simulink model "LaneFollowingNMPC"  (R2021a)
settings: Solver=FixedStepAuto  StartTime=0.0  StopTime=t(end)  FixedStep=Ts  RelTol=1e-3
PreLoadFcn:
  | LaneFollowingUsingNMPCData
values from neighbouring files (symbols this model uses):
  nlobj = nlmpc(7,3,'MV',[1 2],'MD',3,'UD',4)    [LaneFollowingUsingNMPCExample.m]
  phi0 = 0    [CurriculumAngledGetCurvature.m]    (also in DoubleLaneChangeGetCurvature.m; FalconeDoubleLaneChangeGetCurvature.m; FigureEightGetCurvature.m = 1.57079632679; HairpinGetCurvature.m = 1.57079632679)
  Ts = u(5)    [LaneFollowingEKFStateFcn.m]    (also in LaneFollowingUsingNMPCData.m = 0.05; read_csv_model.m = 0.05)
  v0 = v_seq_1.signals.values(1)    [LaneFollowingUsingNMPCData.m]
  v_seq = repelem(Vx, size(Xref, 2))    [FigureEightGetCurvature.m]    (also in LaneFollowingUsingNMPCData.m = v_seq_1.signals.values)
  Xref = [x_initial, Xref(1, 2:end)]    [CurriculumAngledGetCurvature.m]    (also in DoubleLaneChangeGetCurvature.m = Vx*time; FalconeDoubleLaneChangeGetCurvature.m = 0.0:0.05:120; FigureEightGetCurvature.m = A * cos(2. * pi * segments / num_segments); HairpinGetCurvature.m = [Xref, last_arm])
  Yref = [y_initial, Yref(1, 2:end)]    [CurriculumAngledGetCurvature.m]    (also in DoubleLaneChangeGetCurvature.m = 8.1/2*(1+tanh(z1)) - 11.4/2.*(1+tanh(z2)); FalconeDoubleLaneChangeGetCurvature.m = 4.05/2*(1+tanh(z1)) - 5.7/2.*(1+tanh(z2)); FigureEightGetCurvature.m = B * 0.5 * sin(4. * pi * segments / num_segments); HairpinGetCurvature.m = [Yref, last_arm_y])
undefined symbols (not defined in the file or in its folder): DiscIntNeverNeededParam, rho, v_seq_1
libraries: mpcadaslib x1, sharedTrackingLibrary x1, mpclib x1, autolibshared x1
settings Model: NumberOfSteps=3  Creator=The MathWorks, Inc.  LastModifiedBy=sarahaguasvivas
settings SolverCC: AlgebraicLoopSolver=TrustRegion
settings DataIOCC: ReturnWorkspaceOutputs=off
settings DebuggingCC: PregeneratedLibrarySubsystemCodeDiagnostic=none  SFMachineParentedDataDiag=warning  ArithmeticOperatorsInVariantConditions=warning
settings SFSimCC: SimUseLocalCustomCode=off  CustomCodeUndefinedFunction=UseInterfaceOnly
settings RTWCC: RTWUseLocalCustomCode=off
settings CodeAppCC: StateflowObjectComments=on

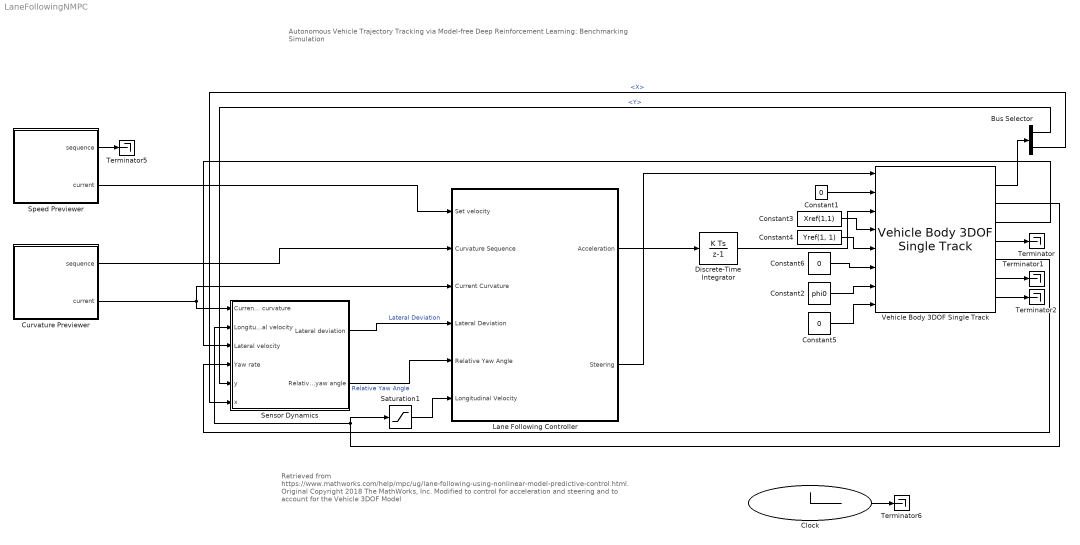
== system LaneFollowingNMPC ==
  note: Retrieved from https://www.mathworks.com/help/mpc/ug/lane-following-using-nonlinear-model-predictive-control.html. Original Copyright 2018 The MathWorks, Inc.
      |
      | Modified to control for acceleration and steering and to account for the Vehicle 3DOF Model
  note: Autonomous Vehicle Trajectory Tracking via Model-free Deep Reinforcement Learning: Benchmarking Simulation
  Bus Selector : BusSelector  OutputSignals=InertFrm.FrntAxl.Disp.Y,InertFrm.FrntAxl.Disp.X
  Clock : Clock
  Constant1 : Constant  Value=0
  Constant2 : Constant  Value=phi0
  Constant3 : Constant  Value=Xref(1,1)
  Constant4 : Constant  Value=Yref(1, 1)
  Constant5 : Constant  Value=0
  Constant6 : Constant  Value=0
  Curvature Previewer : Subsystem  mask{signal=rho, ts=Ts, steps=nlobj.PredictionHorizon}
      mask prompts: signal "Signal name"; ts "Sampling time"; steps "Number of previewing steps"
      mask init:
      | ts = evalin('base',get_param(gcbh,'ts'));
      | signal = evalin('base',get_param(gcbh,'signal'));
      | steps = evalin('base',get_param(gcbh,'steps'));
      | data = mpc_previewer_maskinit(signal,ts);
      mask Display:
      | fprintf('Future\nsample\nextractor');
      | port_label('output', 1, 'seq')
      | port_label('output', 2, '@t')
  Discrete-Time Integrator : DiscreteIntegrator  InitialCondition=v_seq(1)  SampleTime=Ts  LimitOutput=on  UpperSaturationLimit=50  ICPrevOutput=DiscIntNeverNeededParam  ICPrevScaledInput=DiscIntNeverNeededParam
  Lane Following Controller : Subsystem  Variant=on
  Saturation1 : Saturate  UpperLimit=Inf  LowerLimit=1e-5  OutDataTypeStr=double
  Sensor Dynamics : Subsystem
  Speed Previewer : Subsystem  mask{signal=v_seq_1, ts=Ts, steps=1}
      mask prompts: signal "Signal name"; ts "Sampling time"; steps "Number of previewing steps"
      mask init:
      | ts = evalin('base',get_param(gcbh,'ts'));
      | signal = evalin('base',get_param(gcbh,'signal'));
      | steps = evalin('base',get_param(gcbh,'steps'));
      | data = mpc_previewer_maskinit(signal,ts);
      mask Display:
      | fprintf('Future\nsample\nextractor');
      | port_label('output', 1, 'seq')
      | port_label('output', 2, '@t')
  Terminator{,1..2,5..6} (5 alike) : Terminator
  Vehicle Body 3DOF Single Track : autolibshared/Vehicle Body 3DOF Single Track  trackMode=Single (bicycle)  inputMode=External longitudinal velocity  frontSteerMode=on  rearSteerMode=on  windMode=off  muMode=off  extFMode=off  extMMode=off  htchFMode=off  htchMMode=off  extXo=on  extpsio=on  extxdoto=off  extro=on  extYo=on  extTamb=off  extydoto=on  aMode=2  NF=2  NR=2  m=2000  a=1.4  b=1.6  h=0.35  dh=1  hh=0.2  X_o=0  xdot_o=0  CalphaMode=off  sigmaMode=off  d=0  hl=0  w=[1.4,1.4]  Cy_f=19e3  Cy_r=33.5e3  sigma_f=.1  sigma_r=.1  alpha_f_brk=[-.1 .1]  Cy_f_data=[-9e3 9e3]  alpha_r_brk=[-.1 .1]  Cy_r_data=[-9e3 9e3]  Y_o=0  ydot_o=0  Izz=4000  psi_o=0  r_o=0  Af=0  Cd=.0  Cl=.0  Cpm=.0  beta_w=[0:0.01:0.3]  Cs=[0:0.03:0.9]  Cym=[0:0.01:0.3]  Pabs=101325  Tair=273  g=9.81  mu=1.  xdot_tol=.01  Fznom=5000  Fxtire_sat=7e4  Fytire_sat=7e4  longOff=0  latOff=0  vertOff=0  wrapAng=off
      settings: SourceProductBaseCode=PW,DR,MT,UV,VE
  wires:
  Vehicle Body 3DOF Single Track/5 -> Sensor Dynamics/4(Yaw rate)
  Sensor Dynamics/1(Lateral deviation) -> Lane Following Controller/4(Lateral Deviation)  "Lateral Deviation"
  Sensor Dynamics/2(Relative yaw angle) -> Lane Following Controller/5(Relative Yaw Angle)  "Relative Yaw Angle"
  Vehicle Body 3DOF Single Track/6 -> Terminator1/1
  Vehicle Body 3DOF Single Track/7 -> Terminator2/1
  Vehicle Body 3DOF Single Track/1 -> Bus Selector/1
  Vehicle Body 3DOF Single Track/3 -> Sensor Dynamics/3(Lateral velocity)
  Discrete-Time Integrator/1 -> Vehicle Body 3DOF Single Track/3
  Vehicle Body 3DOF Single Track/2 -> Saturation1/1, Sensor Dynamics/2(Longitudinal velocity)
  Speed Previewer/2(current) -> Lane Following Controller/1(Set velocity)
  Saturation1/1 -> Lane Following Controller/6(Longitudinal Velocity)
  Curvature Previewer/2(current) -> Sensor Dynamics/1(Current curvature), Lane Following Controller/3(Current Curvature)
  Constant2/1 -> Vehicle Body 3DOF Single Track/7
  Constant3/1 -> Vehicle Body 3DOF Single Track/4
  Constant4/1 -> Vehicle Body 3DOF Single Track/5
  Constant5/1 -> Vehicle Body 3DOF Single Track/8
  Constant6/1 -> Vehicle Body 3DOF Single Track/6
  Lane Following Controller/1(Acceleration) -> Discrete-Time Integrator/1
  Constant1/1 -> Vehicle Body 3DOF Single Track/2
  Curvature Previewer/1(sequence) -> Lane Following Controller/2(Curvature Sequence)
  Lane Following Controller/2(Steering) -> Vehicle Body 3DOF Single Track/1
  Bus Selector/2 -> Sensor Dynamics/6(x)  "<X>"
  Bus Selector/1 -> Sensor Dynamics/5(y)  "<Y>"
  Speed Previewer/1(sequence) -> Terminator5/1
  Clock/1 -> Terminator6/1
  Vehicle Body 3DOF Single Track/4 -> Terminator/1

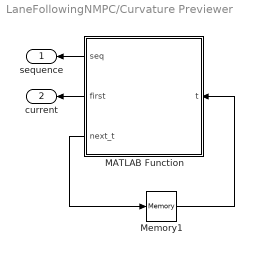
== system LaneFollowingNMPC/Curvature Previewer ==
  MATLAB Function : MATLAB Function  TreatAsAtomicUnit=on
  Memory1 : Memory  InitialCondition=1  InheritSampleTime=on  LinearizeAsDelay=on
  sequence : Outport  VectorParamsAs1DForOutWhenUnconnected=off
  current : Outport  Port=2  VectorParamsAs1DForOutWhenUnconnected=off
  wires:
  MATLAB Function/1(seq) -> sequence/1
  MATLAB Function/2(first) -> current/1
  Memory1/1 -> MATLAB Function/1(t)
  MATLAB Function/3(next_t) -> Memory1/1

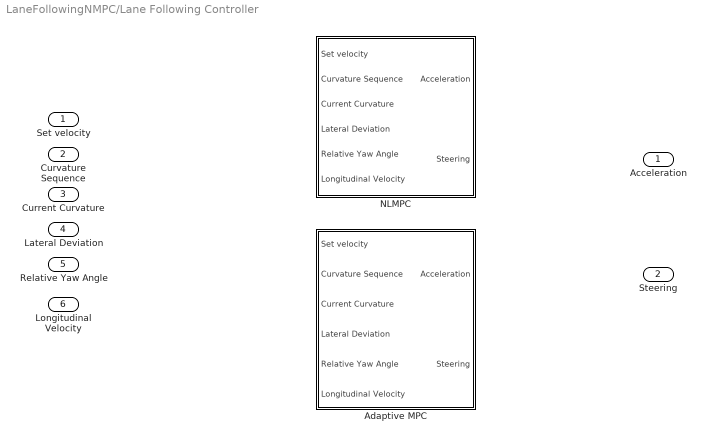
== system LaneFollowingNMPC/Lane Following Controller ==
  Set velocity : Inport
  Curvature Sequence : Inport  Port=2
  Current Curvature : Inport  Port=3
  Lateral Deviation : Inport  Port=4
  Relative Yaw Angle : Inport  Port=5
  Longitudinal Velocity : Inport  Port=6
  Adaptive MPC : Subsystem  VariantControl=controller_type == 2
  NLMPC : Subsystem  VariantControl=controller_type ==1
  Acceleration : Outport  VectorParamsAs1DForOutWhenUnconnected=off
  Steering : Outport  Port=2  VectorParamsAs1DForOutWhenUnconnected=off

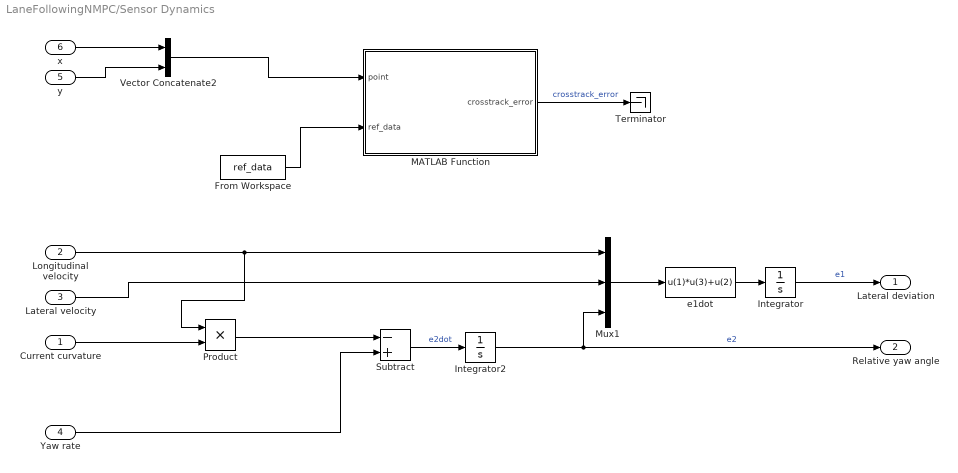
== system LaneFollowingNMPC/Sensor Dynamics ==
  Current curvature : Inport
  Longitudinal velocity : Inport  Port=2
  Lateral velocity : Inport  Port=3
  Yaw rate : Inport  Port=4
  y : Inport  Port=5
  x : Inport  Port=6
  From Workspace : FromWorkspace  VariableName=ref_data
  Integrator : Integrator
  Integrator2 : Integrator
  MATLAB Function : MATLAB Function
  Mux1 : Mux  Inputs=[1 1 1]
  Product : Product
  Subtract : Sum  Inputs=-+
  Terminator : Terminator
  Vector Concatenate2 : Concatenate
  e1dot : Fcn  Expr=u(1)*u(3)+u(2)
  Lateral deviation : Outport  VectorParamsAs1DForOutWhenUnconnected=off
  Relative yaw angle : Outport  Port=2  VectorParamsAs1DForOutWhenUnconnected=off
  wires:
  Current curvature/1 -> Product/2
  Mux1/1 -> e1dot/1
  e1dot/1 -> Integrator/1
  Longitudinal velocity/1 -> Product/1, Mux1/1
  Lateral velocity/1 -> Mux1/2
  Integrator/1 -> Lateral deviation/1  "e1"
  Product/1 -> Subtract/1
  Yaw rate/1 -> Subtract/2
  Subtract/1 -> Integrator2/1  "e2dot"
  Integrator2/1 -> Relative yaw angle/1, Mux1/3  "e2"
  y/1 -> Vector Concatenate2/2
  x/1 -> Vector Concatenate2/1
  MATLAB Function/1(crosstrack_error) -> Terminator/1  "crosstrack_error"
  Vector Concatenate2/1 -> MATLAB Function/1(point)
  From Workspace/1 -> MATLAB Function/2(ref_data)

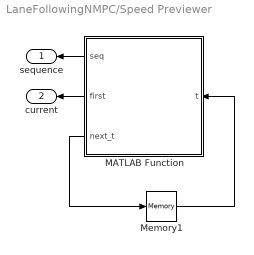
== system LaneFollowingNMPC/Speed Previewer ==
  MATLAB Function : MATLAB Function  TreatAsAtomicUnit=on
  Memory1 : Memory  InitialCondition=1  InheritSampleTime=on  LinearizeAsDelay=on
  sequence : Outport  VectorParamsAs1DForOutWhenUnconnected=off
  current : Outport  Port=2  VectorParamsAs1DForOutWhenUnconnected=off
  wires:
  MATLAB Function/1(seq) -> sequence/1
  MATLAB Function/2(first) -> current/1
  Memory1/1 -> MATLAB Function/1(t)
  MATLAB Function/3(next_t) -> Memory1/1

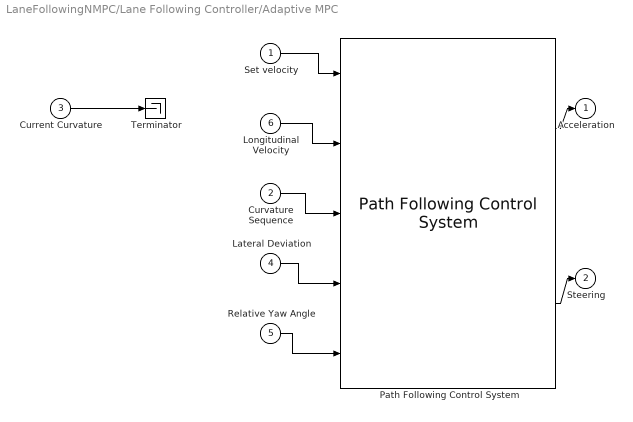
== system LaneFollowingNMPC/Lane Following Controller/Adaptive MPC ==
  Set velocity : Inport
  Curvature Sequence : Inport  Port=2
  Current Curvature : Inport  Port=3
  Lateral Deviation : Inport  Port=4
  Relative Yaw Angle : Inport  Port=5
  Longitudinal Velocity : Inport  Port=6
  Path Following Control System : mpcadaslib/Path Following Control System  VariantControl=Variant2  ModelType=Use vehicle parameters  VehicleMass=m  VehicleYawInertia=Iz  LengthToFront=lf  LengthToRear=lr  FrontTireStiffness=Cf  RearTireStiffness=Cr  AccelTimeConstant=tau  EgoModelMatrixA=[-2,zeros(1,3);1,zeros(1,3);zeros(1,2),-4.4021,-12.4603;zeros(1,2),1.3913,-5.1868]  EgoModelMatrixB=[2,zeros(1,3);zeros(1,2),24.1270,15.8609]'  EgoModelMatrixC=[zeros(3,1),eye(3)]  InitialLongVel=v_seq(1)  TransportLag=0  spaceCtrl=off  DefaultSpacing=10  MinSteering=-1.13  umin_ext=off  MaxSteering=1.13  umax_ext=off  MinAcceleration=-26.5  amin_ext=off  MaxAcceleration=6.  amax_ext=off  Ts=Ts  PredictionHorizon=nlobj.PredictionHorizon  ControlHorizon=nlobj.ControlHorizon  LongWeight=1  LateralWeight=1  AccelRateWeight=0.3  SteerRateWeight=0.3  suboptimal=off  maxiter=10  datatypeopt=double  optmode=off  trackmode=off
      settings: SourceProductBaseCode=MP
  Terminator : Terminator
  Acceleration : Outport  VectorParamsAs1DForOutWhenUnconnected=off
  Steering : Outport  Port=2  VectorParamsAs1DForOutWhenUnconnected=off
  wires:
  Current Curvature/1 -> Terminator/1
  Path Following Control System/2 -> Steering/1
  Path Following Control System/1 -> Acceleration/1
  Set velocity/1 -> Path Following Control System/1
  Longitudinal Velocity/1 -> Path Following Control System/2
  Curvature Sequence/1 -> Path Following Control System/3
  Lateral Deviation/1 -> Path Following Control System/4
  Relative Yaw Angle/1 -> Path Following Control System/5

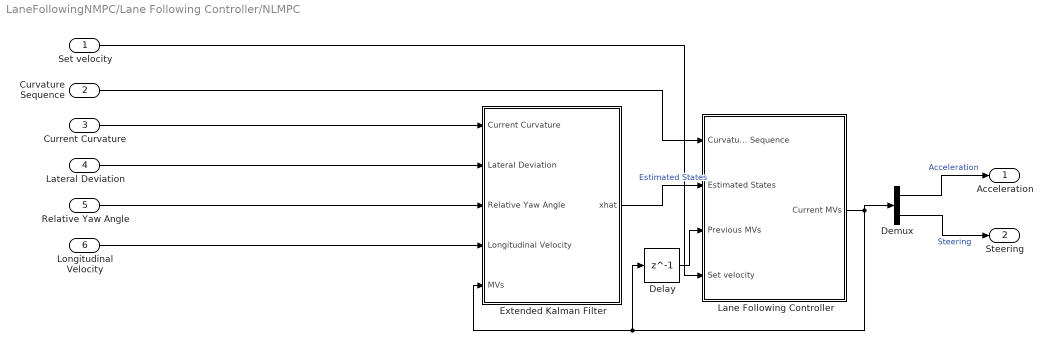
== system LaneFollowingNMPC/Lane Following Controller/NLMPC ==
  Set velocity : Inport
  Curvature Sequence : Inport  Port=2
  Current Curvature : Inport  Port=3
  Lateral Deviation : Inport  Port=4
  Relative Yaw Angle : Inport  Port=5
  Longitudinal Velocity : Inport  Port=6
  Delay : Delay  DelayLength=1  InitialCondition=[0.2 0.3]
  Demux : Demux  Outputs=2
  Extended Kalman Filter : Subsystem
  Lane Following Controller : Subsystem
  Acceleration : Outport  VectorParamsAs1DForOutWhenUnconnected=off
  Steering : Outport  Port=2  VectorParamsAs1DForOutWhenUnconnected=off
  wires:
  Extended Kalman Filter/1(xhat) -> Lane Following Controller/2(Estimated States)  "Estimated States"
  Lane Following Controller/1(Current MVs) -> Demux/1, Extended Kalman Filter/5(MVs), Delay/1
  Lateral Deviation/1 -> Extended Kalman Filter/2(Lateral Deviation)
  Curvature Sequence/1 -> Lane Following Controller/1(Curvature Sequence)
  Longitudinal Velocity/1 -> Extended Kalman Filter/4(Longitudinal Velocity)
  Delay/1 -> Lane Following Controller/3(Previous MVs)
  Relative Yaw Angle/1 -> Extended Kalman Filter/3(Relative Yaw Angle)
  Current Curvature/1 -> Extended Kalman Filter/1(Current Curvature)
  Set velocity/1 -> Lane Following Controller/4(Set velocity)
  Demux/2 -> Steering/1  "Steering"
  Demux/1 -> Acceleration/1  "Acceleration"

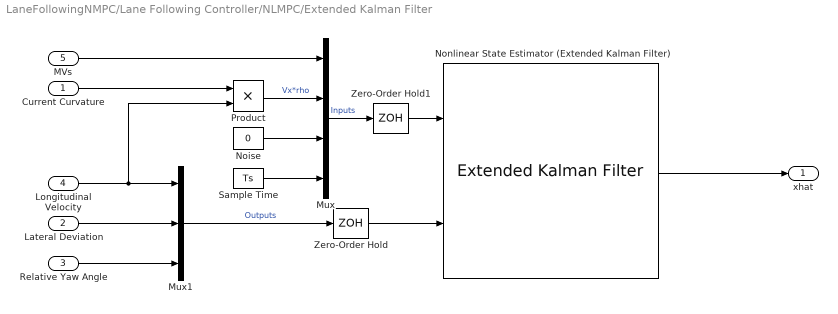
== system LaneFollowingNMPC/Lane Following Controller/NLMPC/Extended Kalman Filter ==
  Current Curvature : Inport
  Lateral Deviation : Inport  Port=2
  Relative Yaw Angle : Inport  Port=3
  Longitudinal Velocity : Inport  Port=4
  MVs : Inport  Port=5
  Mux : Mux
  Mux1 : Mux  Inputs=3
  Noise : Constant  Value=0
  Nonlinear State Estimator (Extended Kalman Filter) : sharedTrackingLibrary/Extended Kalman Filter  StateTransitionFcn=LaneFollowingEKFStateFcn  HasStateTransitionJacobianFcn=off  HasAdditiveProcessNoise=Additive  ProcessNoise=1e-4*eye(7)  HasTimeVaryingProcessNoise=off  HasStateTransitionFcnExtraArgument=1  InitialState=[0 0 v0 0 0 0 0]'  InitialStateCovariance=1e-4*eye(7)  MeasurementFcn1=LaneFollowingEKFMeasFcn  HasMeasurementJacobianFcn1=off  HasMeasurementEnablePort1=off  HasAdditiveMeasurementNoise1=Additive  MeasurementNoise1=1e-4*eye(3)  HasTimeVaryingMeasurementNoise1=off  HasMeasurementFcnExtraArgument1=0  MeasurementFcn2=myMeasurementFcn  HasMeasurementJacobianFcn2=off  HasMeasurementEnablePort2=off  HasAdditiveMeasurementNoise2=Additive  MeasurementNoise2=1  HasTimeVaryingMeasurementNoise2=off  HasMeasurementFcnExtraArgument2=0  MeasurementFcn3=myMeasurementFcn  HasMeasurementJacobianFcn3=off  HasMeasurementEnablePort3=off  HasAdditiveMeasurementNoise3=Additive  MeasurementNoise3=1  HasTimeVaryingMeasurementNoise3=off  HasMeasurementFcnExtraArgument3=0  MeasurementFcn4=myMeasurementFcn  HasMeasurementJacobianFcn4=off  HasMeasurementEnablePort4=off  HasAdditiveMeasurementNoise4=Additive  MeasurementNoise4=1  HasTimeVaryingMeasurementNoise4=off  HasMeasurementFcnExtraArgument4=0  MeasurementFcn5=myMeasurementFcn  HasMeasurementJacobianFcn5=off  HasMeasurementEnablePort5=off  HasAdditiveMeasurementNoise5=Additive  MeasurementNoise5=1  HasTimeVaryingMeasurementNoise5=off  HasMeasurementFcnExtraArgument5=0  EnableMultirate=off  StateTransitionFcnSampleTime=1  MeasurementFcn1SampleTime=1  MeasurementFcn2SampleTime=1  MeasurementFcn3SampleTime=1  MeasurementFcn4SampleTime=1  MeasurementFcn5SampleTime=1  UseCurrentEstimator=on  OutputStateCovariance=off  DataType=double  SampleTime=Ts  NumberOfMeasurements=1
      settings: SourceProductBaseCode=CT,DR,TF,ID,LP,NV,AR,RO,RR,UV,VE
  Product : Product
  Sample Time : Constant  Value=Ts
  Zero-Order Hold : ZeroOrderHold  SampleTime=Ts
  Zero-Order Hold1 : ZeroOrderHold  SampleTime=Ts
  xhat : Outport  VectorParamsAs1DForOutWhenUnconnected=off
  wires:
  Noise/1 -> Mux/3
  Zero-Order Hold/1 -> Nonlinear State Estimator (Extended Kalman Filter)/2
  MVs/1 -> Mux/1
  Sample Time/1 -> Mux/4
  Nonlinear State Estimator (Extended Kalman Filter)/1 -> xhat/1
  Mux1/1 -> Zero-Order Hold/1  "Outputs"
  Lateral Deviation/1 -> Mux1/2
  Longitudinal Velocity/1 -> Mux1/1, Product/2
  Relative Yaw Angle/1 -> Mux1/3
  Current Curvature/1 -> Product/1
  Product/1 -> Mux/2  "Vx*rho"
  Mux/1 -> Zero-Order Hold1/1  "Inputs"
  Zero-Order Hold1/1 -> Nonlinear State Estimator (Extended Kalman Filter)/1

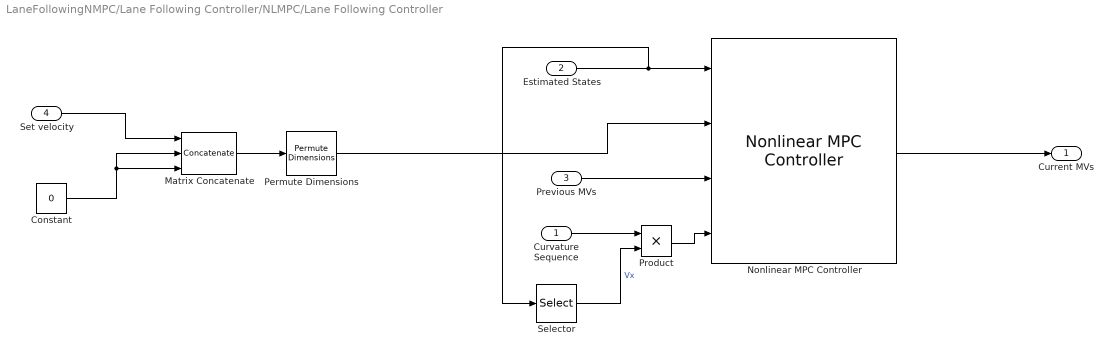
== system LaneFollowingNMPC/Lane Following Controller/NLMPC/Lane Following Controller ==
  Curvature Sequence : Inport
  Estimated States : Inport  Port=2
  Previous MVs : Inport  Port=3
  Set velocity : Inport  Port=4
  Constant : Constant  Value=0
  Matrix Concatenate : Concatenate  NumInputs=3  ConcatenateDimension=2
  Nonlinear MPC Controller : mpclib/Nonlinear MPC Controller  SCDEnableBlockLinearizationSpecification=on  nlmpcobj=nlobj  UseObjectTs=off  TsControl=Ts  UseMEX=off  md_enabled=on  mvtarget_enabled=off  param_enabled=off  cost_enabled=off  mvseq_enabled=off  stateseq_enabled=off  ovseq_enabled=off  slack_enabled=off  status_enabled=off  ov_min=off  ov_max=off  mv_min=off  mv_max=off  mvrate_min=off  mvrate_max=off  state_min=off  state_max=off  ov_weight=off  mv_weight=off  mvrate_weight=off  ecr_weight=off  nlp_initialize=off
      settings: SourceProductName=Model Predictive Control Toolbox
  Permute Dimensions : PermuteDimensions
  Product : Product
  Selector : Selector  InputPortWidth=7  IndexOptions=Index vector (dialog)  Indices=[3]  OutputSizes=1
  Current MVs : Outport  VectorParamsAs1DForOutWhenUnconnected=off
  wires:
  Previous MVs/1 -> Nonlinear MPC Controller/3
  Estimated States/1 -> Selector/1, Nonlinear MPC Controller/1
  Nonlinear MPC Controller/1 -> Current MVs/1
  Selector/1 -> Product/2  "Vx"
  Curvature Sequence/1 -> Product/1
  Product/1 -> Nonlinear MPC Controller/4
  Set velocity/1 -> Matrix Concatenate/1
  Constant/1 -> Matrix Concatenate/2, Matrix Concatenate/3
  Permute Dimensions/1 -> Nonlinear MPC Controller/2
  Matrix Concatenate/1 -> Permute Dimensions/1

== matlab function LaneFollowingNMPC/Curvature Previewer/MATLAB Function ==
  settings: updateMethod=DISCRETE  sampleTime=ts
  data: data parameter; seq output; steps parameter; t input; first output; next_t output
function [seq,first,next_t] = fcn(data,steps,t)
%#codegen
[seq,first,next_t] = mpcblock_preview('md',data,steps,t);

== matlab function LaneFollowingNMPC/Speed Previewer/MATLAB Function ==
  settings: updateMethod=DISCRETE  sampleTime=ts
  data: data parameter; seq output; steps parameter; t input; first output; next_t output
function [seq,first,next_t] = fcn(data,steps,t)
%#codegen
[seq,first,next_t] = mpcblock_preview('md',data,steps,t);

== matlab function LaneFollowingNMPC/Sensor Dynamics/MATLAB Function ==
  data: point input double size=[1, 2]; crosstrack_error output double size=1; ref_data input double size=[size(Xref, 2), 2]
function crosstrack_error  = fcn(point, ref_data)
    crosstrack_error = 0.0;
    dist = zeros(size(ref_data, 1), 1);
    for i = 1:length(ref_data)
        dist(i, 1) = pdist([point; ref_data(i, :)], 'Euclidean');
    end
    crosstrack_error = min(dist);
end
